simulink library "simiam"  (Simulink 8.0)
settings: Solver=ode45  StartTime=0.0  StopTime=10.0  RelTol=1e-3
values from neighbouring files (symbols this model uses):
  thetai = 0    [param.m]
  xi = 0    [param.m]
  yi = 0    [param.m]
settings Model: Creator=jdelacroix  LastModifiedBy=samati

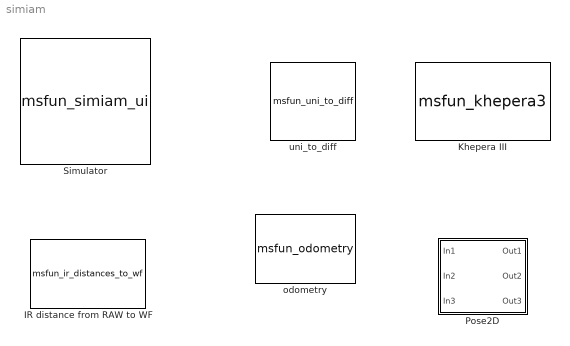
== system simiam ==
  IR distance from RAW to WF : M-S-Function  FunctionName=msfun_ir_distances_to_wf
      mask Display:
      | port_label('input', 1, 'x')
      | port_label('input', 2, 'y')
      | port_label('input', 3, 'theta')
      | port_label('input', 4, 'ir_raw')
      | port_label('output', 1, 'ir_wf')
  Khepera III : M-S-Function  FunctionName=msfun_khepera3  Parameters=x_0,y_0,theta_0  mask(Khepera3){x_0=0, y_0=0, theta_0=0, robot_id=1}
      mask prompts: robot_id "ID"
      mask Display:
      | port_label('output', 1, 'ir_raw')
      | port_label('output', 2, 'wheel_ticks')
      | port_label('input', 1, 'vel_r')
      | port_label('input', 2, 'vel_l')
  Pose2D : Subsystem
      mask Display:
      | port_label('input', 1, 'x')
      | port_label('input', 2, 'y')
      | port_label('input', 3, 'theta')
      | port_label('output', 1, 'x')
      | port_label('output', 2, 'y')
      | port_label('output', 3, 'theta')
  Simulator : M-S-Function  FunctionName=msfun_simiam_ui  mask(Simulator){}
      mask Display: image(imread('simulink/simiam-round-logo.png'))
  odometry : M-S-Function  FunctionName=msfun_odometry  Parameters=wheel_radius,wheel_base_length,ticks_per_rev  mask{wheel_radius=0.021, wheel_base_length=0.0885, ticks_per_rev=2675}
      mask Display:
      | port_label('input', 1, 'x')
      | port_label('input', 2, 'y')
      | port_label('input', 3, 'theta')
      | port_label('input', 4, 'wheel_ticks')
      | port_label('output', 1, 'x')
      | port_label('output', 2, 'y')
      | port_label('output', 3, 'theta')
  uni_to_diff : M-S-Function  FunctionName=msfun_uni_to_diff  Parameters=wheel_radius,wheel_base_length  mask{wheel_radius=0.021, wheel_base_length=0.0885}
      mask Display:
      | port_label('output', 1, 'vel_r')
      | port_label('output', 2, 'vel_l')
      | port_label('input', 1, 'v')
      | port_label('input', 2, 'w')

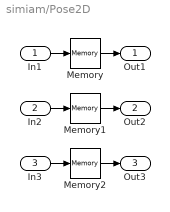
== system simiam/Pose2D ==
  In1 : Inport
  In2 : Inport  Port=2
  In3 : Inport  Port=3
  Memory : Memory  X0=xi  InheritSampleTime=on  StateIdentifier=state_estimate_x
  Memory1 : Memory  X0=yi  InheritSampleTime=on  StateIdentifier=state_estimate_y
  Memory2 : Memory  X0=thetai  InheritSampleTime=on  StateIdentifier=state_estimate_theta
  Out1 : Outport
  Out2 : Outport  Port=2
  Out3 : Outport  Port=3
  wires:
  In3/1 -> Memory2/1
  Memory1/1 -> Out2/1
  In1/1 -> Memory/1
  Memory/1 -> Out1/1
  Memory2/1 -> Out3/1
  In2/1 -> Memory1/1
